simulink model "PID_time_scale_sep"  (R2023b)
settings: Solver=VariableStepAuto  StartTime=0.0  StopTime=2000  RelTol=1e-3
values from neighbouring files (symbols this model uses):
  beta = 40*pi/180    (= 0.698131700798)    [init_PID_time_scale_sep.m]
  H_c_max = 0.035    [init_PID_time_scale_sep.m]
  I = [2.10, 0, 0; 0, 2.3, -0.03; 0.01, -0.03, 1.72]    [init_PID_time_scale_sep.m]
  I_inv = inv(I)    [init_PID_time_scale_sep.m]
  K_redist = [1;1;5]*1e0    [init_PID_time_scale_sep.m]
  K_unload = 1.5*[1;1;1]*1e2    [init_PID_time_scale_sep.m]
  Kd_t = 2*1e-4    (= 0.0002)    [init_PID_time_scale_sep.m]
  Kd_w = 1e-1    (= 0.1)    [init_PID_time_scale_sep.m]
  Ki_t = [1;1;10]*1e-8    [init_PID_time_scale_sep.m]
  Ki_w = 0  *1e-4    (= 0)    [init_PID_time_scale_sep.m]
  Kp_t = [1;1;1]*1e-2    [init_PID_time_scale_sep.m]
  Kp_w = 1.1*[1;1 ;1]*1e-1    [init_PID_time_scale_sep.m]
  n = sqrt(mu/R^3)    [init_PID_time_scale_sep.m]
  Omega_des = [0.2,0.2,0.2].'*pi/180*0    [init_PID_time_scale_sep.m]
  Omega_i = [15    , -15, 15].'*pi/180    [init_PID_time_scale_sep.m]
  p1 = pi    (= 3.14159265359)    [init_PID_time_scale_sep.m]
  p2 = pi/2    (= 1.57079632679)    [init_PID_time_scale_sep.m]
  p3 = pi/4    (= 0.785398163397)    [init_PID_time_scale_sep.m]
  R_rw = [cos(beta), 0, -cos(beta), 0 ... (first row only)    [init_PID_time_scale_sep.m]
  R_rw_pinv = pinv(R_rw)    [init_PID_time_scale_sep.m]
  T_c_max = 0.015    [init_PID_time_scale_sep.m]
  T_d = 1e-6    (= 1e-06)    [init_PID_time_scale_sep.m]
  Theta_des = [30,50,70].'*pi/180    [init_PID_time_scale_sep.m]
  Theta_i = [0,0,0].'    [init_PID_time_scale_sep.m]
libraries: matrix_library x2
settings Model: Creator=subhechha  LastModifiedBy=subhechha

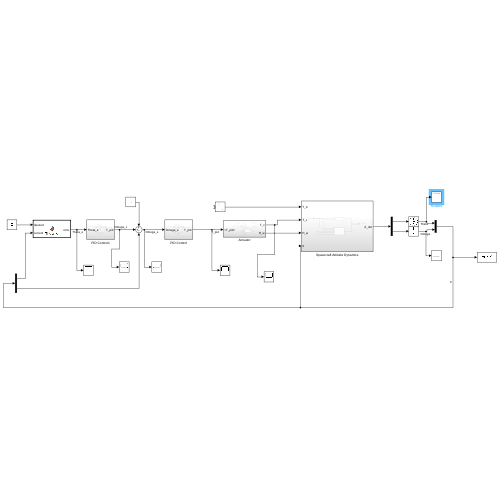
[thumbnail: Simulink's stored preview of the top-level diagram]
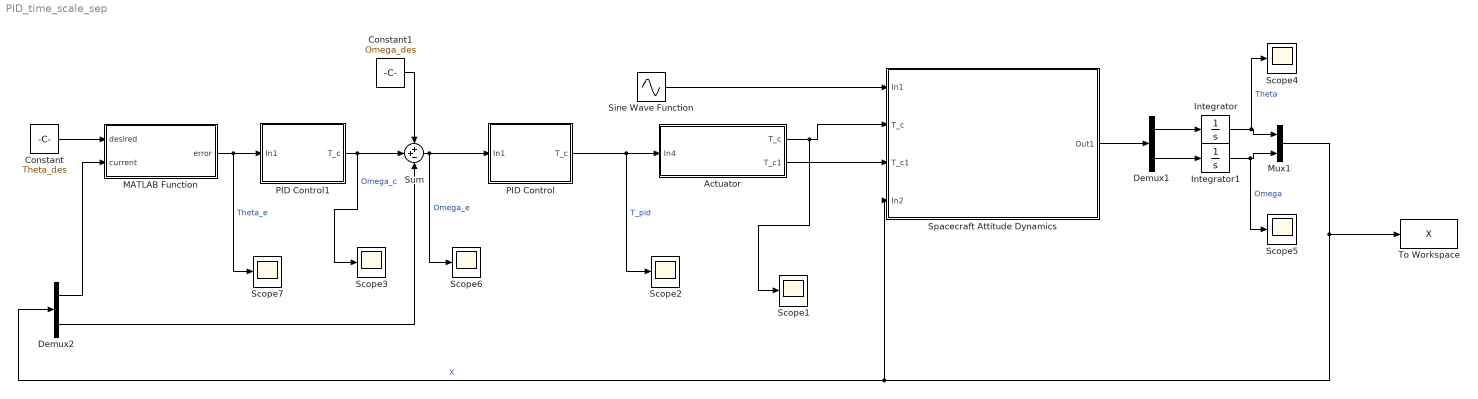
== system PID_time_scale_sep ==
  Actuator : Subsystem
  Constant : Constant  Value=Theta_des  VectorParams1D=off
  Constant1 : Constant  Value=Omega_des  VectorParams1D=off
  Demux1 : Demux  Outputs=[3 3]
  Demux2 : Demux  Outputs=[3 3]
  Integrator : Integrator  InitialCondition=Theta_i  WrapState=on  ZeroCross=off
  Integrator1 : Integrator  InitialCondition=Omega_i  ZeroCross=off
  MATLAB Function : MATLAB Function  TreatAsAtomicUnit=on
  Mux1 : Mux  Inputs=[3 3]
  PID Control : Subsystem
  PID Control1 : Subsystem
  Scope{1..7} (7 alike) : Scope
  Sine Wave Function : Sin  TimeSource=Use external signal  Amplitude=[T_d;T_d;T_d]  Frequency=0.01  Phase=[p1;p2;p3]  SampleTime=0
  Spacecraft Attitude Dynamics : Subsystem
  Sum : Sum  Inputs=++-
  To Workspace : ToWorkspace  VariableName=X  SaveFormat=Timeseries  SampleTime=-1
  wires:
  Sum/1 -> PID Control/1(In1), Scope6/1  "Omega_e"
  Actuator/1(T_c) -> Scope1/1, Spacecraft Attitude Dynamics/2(T_c)
  Actuator/2(T_c1) -> Spacecraft Attitude Dynamics/3(T_c1)
  PID Control/1(T_c) -> Scope2/1, Actuator/1(In4)  "T_pid"
  Sine Wave Function/1 -> Spacecraft Attitude Dynamics/1(In1)
  Demux1/2 -> Integrator1/1
  Demux1/1 -> Integrator/1
  Spacecraft Attitude Dynamics/1(Out1) -> Demux1/1
  Mux1/1 -> Demux2/1, Spacecraft Attitude Dynamics/4(In2), To Workspace/1  "X"
  Integrator1/1 -> Scope5/1, Mux1/2  "Omega"
  Integrator/1 -> Scope4/1, Mux1/1  "Theta"
  Demux2/2 -> Sum/3
  PID Control1/1(T_c) -> Sum/2, Scope3/1  "Omega_c"
  MATLAB Function/1(error) -> Scope7/1, PID Control1/1(In1)  "Theta_e"
  Demux2/1 -> MATLAB Function/2(current)
  Constant/1 -> MATLAB Function/1(desired)
  Constant1/1 -> Sum/1

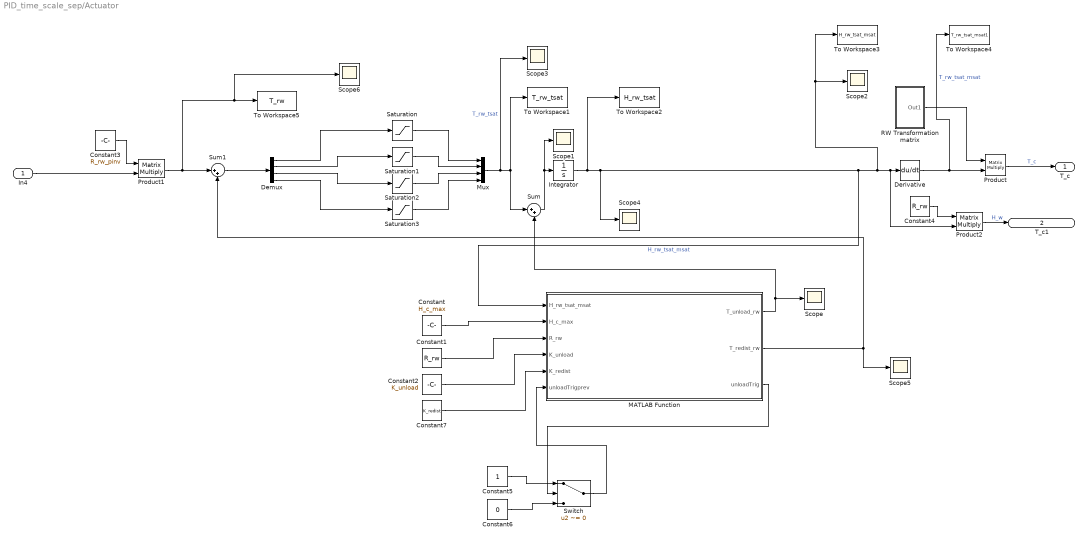
== system PID_time_scale_sep/Actuator ==
  In4 : Inport
  Constant : Constant  Value=H_c_max
  Constant1 : Constant  Value=R_rw  VectorParams1D=off
  Constant2 : Constant  Value=K_unload  VectorParams1D=off
  Constant3 : Constant  Value=R_rw_pinv  VectorParams1D=off
  Constant4 : Constant  Value=R_rw  VectorParams1D=off
  Constant5 : Constant
  Constant6 : Constant  Value=0
  Constant7 : Constant  Value=K_redist  VectorParams1D=off
  Demux : Demux
  Derivative : Derivative
  Integrator : Integrator  LimitOutput=on  UpperSaturationLimit=H_c_max  LowerSaturationLimit=-H_c_max  ZeroCross=off
  MATLAB Function : MATLAB Function  TreatAsAtomicUnit=on
  Mux : Mux
  Product : Product  Multiplication=Matrix(*)
  Product1 : Product  Multiplication=Matrix(*)
  Product2 : Product  Multiplication=Matrix(*)
  RW Transformation matrix : Subsystem
  Saturation{,1..3} (4 alike) : Saturate  UpperLimit=T_c_max  LowerLimit=-T_c_max  LinearizeAsGain=off  ZeroCross=off
  Scope{,1..6} (7 alike) : Scope
  Sum : Sum  Inputs=|++
  Sum1 : Sum  Inputs=|++
  Switch : Switch  Criteria=u2 ~= 0  SaturateOnIntegerOverflow=off  InputSameDT=off
  To Workspace1 : ToWorkspace  VariableName=T_rw_tsat  SaveFormat=Timeseries  SampleTime=-1
  To Workspace2 : ToWorkspace  VariableName=H_rw_tsat  SaveFormat=Timeseries  SampleTime=-1
  To Workspace3 : ToWorkspace  VariableName=H_rw_tsat_msat  SaveFormat=Timeseries  SampleTime=-1
  To Workspace4 : ToWorkspace  VariableName=T_rw_tsat_msat1  SaveFormat=Timeseries  SampleTime=-1
  To Workspace5 : ToWorkspace  VariableName=T_rw  SaveFormat=Timeseries  SampleTime=-1
  T_c : Outport
  T_c1 : Outport  Port=2
  wires:
  Mux/1 -> Scope3/1, To Workspace1/1, Sum/1  "T_rw_tsat"
  Demux/3 -> Saturation2/1
  Demux/2 -> Saturation1/1
  Saturation/1 -> Mux/1
  Saturation3/1 -> Mux/4
  Integrator/1 -> To Workspace2/1, MATLAB Function/1(H_rw_tsat_msat), Product2/2, Derivative/1, Scope2/1, To Workspace3/1, Scope4/1  "H_rw_tsat_msat"
  Saturation1/1 -> Mux/2
  Product1/1 -> Sum1/1, Scope6/1, To Workspace5/1
  Saturation2/1 -> Mux/3
  Demux/1 -> Saturation/1
  Derivative/1 -> To Workspace4/1, Product/2  "T_rw_tsat_msat"
  Demux/4 -> Saturation3/1
  RW Transformation matrix/1(Out1) -> Product/1
  Product/1 -> T_c/1  "T_c"
  Constant/1 -> MATLAB Function/2(H_c_max)
  Constant1/1 -> MATLAB Function/3(R_rw)
  Constant2/1 -> MATLAB Function/4(K_unload)
  In4/1 -> Product1/2
  Constant3/1 -> Product1/1
  Sum/1 -> Scope1/1, Integrator/1
  MATLAB Function/1(T_unload_rw) -> Sum/2, Scope/1
  Product2/1 -> T_c1/1  "H_w"
  Constant4/1 -> Product2/1
  MATLAB Function/3(unloadTrig) -> Switch/2
  Switch/1 -> MATLAB Function/6(unloadTrigprev)
  Constant5/1 -> Switch/1
  Constant6/1 -> Switch/3
  Constant7/1 -> MATLAB Function/5(K_redist)
  MATLAB Function/2(T_redist_rw) -> Sum1/2, Scope5/1
  Sum1/1 -> Demux/1

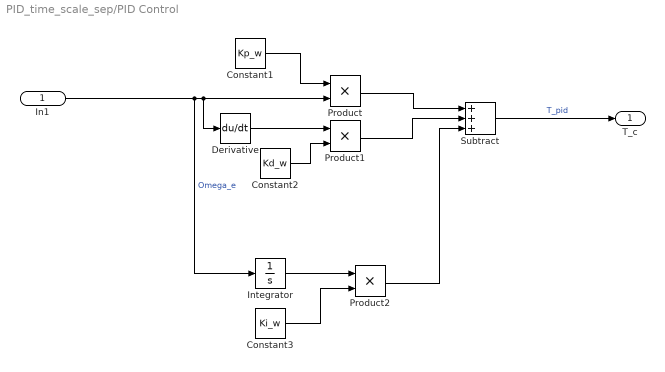
== system PID_time_scale_sep/PID Control ==
  In1 : Inport
  Constant1 : Constant  Value=Kp_w  VectorParams1D=off
  Constant2 : Constant  Value=Kd_w  VectorParams1D=off
  Constant3 : Constant  Value=Ki_w  VectorParams1D=off
  Derivative : Derivative
  Integrator : Integrator  WrapState=on
  Product : Product
  Product1 : Product
  Product2 : Product
  Subtract : Sum  Inputs=+++
  T_c : Outport
  wires:
  Constant2/1 -> Product1/2
  Product1/1 -> Subtract/2
  Constant1/1 -> Product/1
  Product/1 -> Subtract/1
  Subtract/1 -> T_c/1  "T_pid"
  Integrator/1 -> Product2/1
  Constant3/1 -> Product2/2
  Product2/1 -> Subtract/3
  In1/1 -> Integrator/1, Derivative/1, Product/2  "Omega_e"
  Derivative/1 -> Product1/1

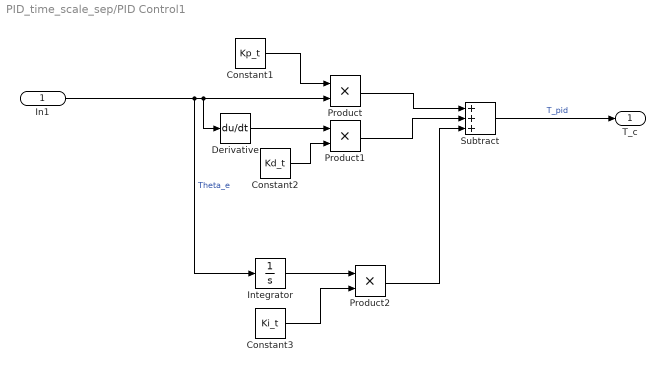
== system PID_time_scale_sep/PID Control1 ==
  In1 : Inport
  Constant1 : Constant  Value=Kp_t  VectorParams1D=off
  Constant2 : Constant  Value=Kd_t  VectorParams1D=off
  Constant3 : Constant  Value=Ki_t  VectorParams1D=off
  Derivative : Derivative
  Integrator : Integrator  WrapState=on
  Product : Product
  Product1 : Product
  Product2 : Product
  Subtract : Sum  Inputs=+++
  T_c : Outport
  wires:
  Constant2/1 -> Product1/2
  Product1/1 -> Subtract/2
  Constant1/1 -> Product/1
  Product/1 -> Subtract/1
  Subtract/1 -> T_c/1  "T_pid"
  Integrator/1 -> Product2/1
  Constant3/1 -> Product2/2
  Product2/1 -> Subtract/3
  In1/1 -> Integrator/1, Derivative/1, Product/2  "Theta_e"
  Derivative/1 -> Product1/1

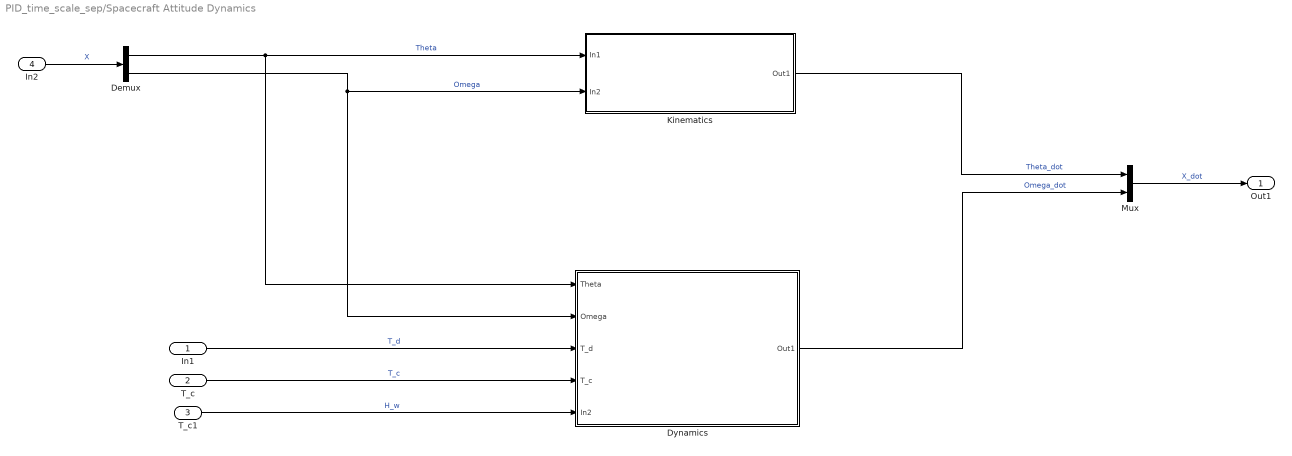
== system PID_time_scale_sep/Spacecraft Attitude Dynamics ==
  In1 : Inport
  T_c : Inport  Port=2
  T_c1 : Inport  Port=3
  In2 : Inport  Port=4
  Demux : Demux  Outputs=[3 3]
  Dynamics : Subsystem
  Kinematics : Subsystem
  Mux : Mux  Inputs=[3 3]
  Out1 : Outport
  wires:
  Dynamics/1(Out1) -> Mux/2  "Omega_dot"
  Kinematics/1(Out1) -> Mux/1  "Theta_dot"
  Demux/1 -> Dynamics/1(Theta), Kinematics/1(In1)  "Theta"
  In1/1 -> Dynamics/3(T_d)  "T_d"
  Demux/2 -> Dynamics/2(Omega), Kinematics/2(In2)  "Omega"
  In2/1 -> Demux/1  "X"
  Mux/1 -> Out1/1  "X_dot"
  T_c/1 -> Dynamics/4(T_c)  "T_c"
  T_c1/1 -> Dynamics/5(In2)  "H_w"

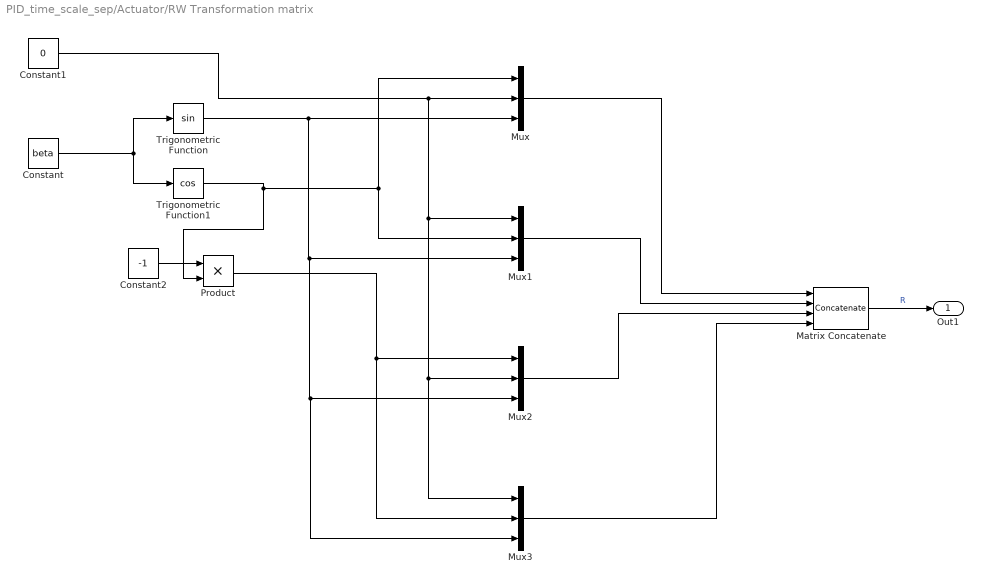
== system PID_time_scale_sep/Actuator/RW Transformation matrix ==
  Constant : Constant  Value=beta
  Constant1 : Constant  Value=0
  Constant2 : Constant  Value=-1
  Matrix Concatenate : Concatenate  NumInputs=4  Mode=Multidimensional array  ConcatenateDimension=2
  Mux{,1..3} (4 alike) : Mux  Inputs=3
  Product : Product
  Trigonometric Function : Trigonometry
  Trigonometric Function1 : Trigonometry  Operator=cos
  Out1 : Outport
  wires:
  Mux3/1 -> Matrix Concatenate/4
  Constant2/1 -> Product/1
  Product/1 -> Mux3/2, Mux2/1
  Mux/1 -> Matrix Concatenate/1
  Trigonometric Function1/1 -> Mux/1, Mux1/2, Product/2
  Mux1/1 -> Matrix Concatenate/2
  Mux2/1 -> Matrix Concatenate/3
  Constant/1 -> Trigonometric Function1/1, Trigonometric Function/1
  Trigonometric Function/1 -> Mux3/3, Mux2/3, Mux1/3, Mux/3
  Constant1/1 -> Mux3/1, Mux2/2, Mux1/1, Mux/2
  Matrix Concatenate/1 -> Out1/1  "R"

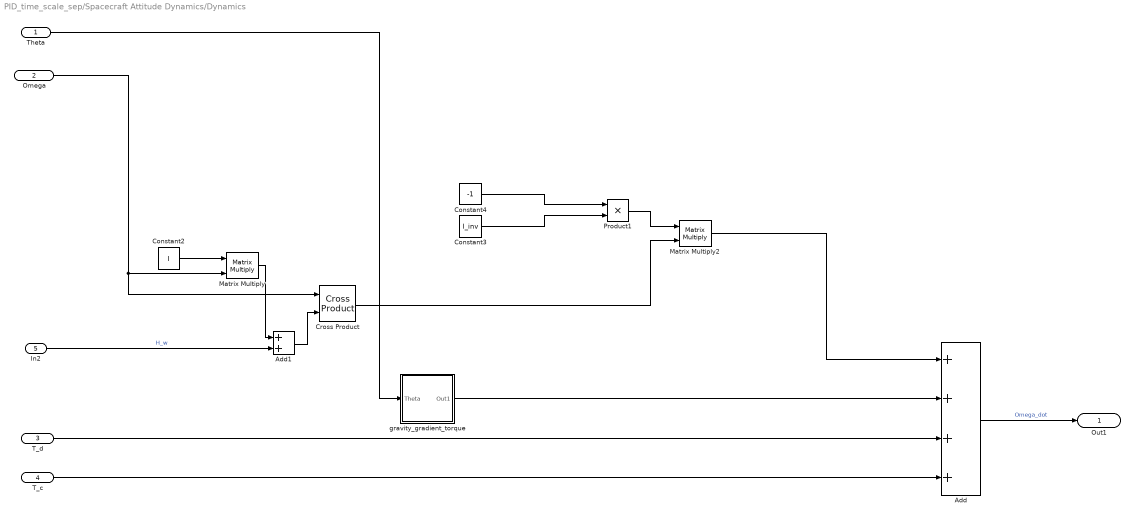
== system PID_time_scale_sep/Spacecraft Attitude Dynamics/Dynamics ==
  Theta : Inport
  Omega : Inport  Port=2
  T_d : Inport  Port=3
  T_c : Inport  Port=4
  In2 : Inport  Port=5
  Add : Sum  Inputs=++++
  Add1 : Sum
  Constant2 : Constant  Value=I  VectorParams1D=off
  Constant3 : Constant  Value=I_inv  VectorParams1D=off
  Constant4 : Constant  Value=-1
  Cross Product : matrix_library/Cross Product
  Matrix Multiply : Product  Multiplication=Matrix(*)
  Matrix Multiply2 : Product  Multiplication=Matrix(*)
  Product1 : Product
  gravity_gradient_torque : Subsystem
  Out1 : Outport
  wires:
  Add/1 -> Out1/1  "Omega_dot"
  T_c/1 -> Add/4
  Matrix Multiply/1 -> Add1/1
  T_d/1 -> Add/3
  Theta/1 -> gravity_gradient_torque/1(Theta)
  Constant4/1 -> Product1/1
  Matrix Multiply2/1 -> Add/1
  Product1/1 -> Matrix Multiply2/1
  Constant2/1 -> Matrix Multiply/1
  Constant3/1 -> Product1/2
  Cross Product/1 -> Matrix Multiply2/2
  Omega/1 -> Cross Product/1, Matrix Multiply/2
  gravity_gradient_torque/1(Out1) -> Add/2
  In2/1 -> Add1/2  "H_w"
  Add1/1 -> Cross Product/2

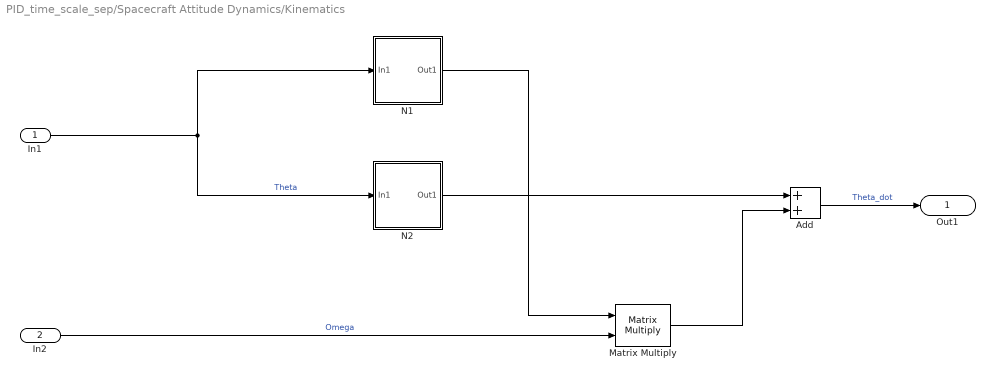
== system PID_time_scale_sep/Spacecraft Attitude Dynamics/Kinematics ==
  In1 : Inport
  In2 : Inport  Port=2
  Add : Sum
  Matrix Multiply : Product  Multiplication=Matrix(*)
  N1 : Subsystem
  N2 : Subsystem
  Out1 : Outport
  wires:
  N2/1(Out1) -> Add/1
  In1/1 -> N1/1(In1), N2/1(In1)  "Theta"
  Matrix Multiply/1 -> Add/2
  N1/1(Out1) -> Matrix Multiply/1
  Add/1 -> Out1/1  "Theta_dot"
  In2/1 -> Matrix Multiply/2  "Omega"

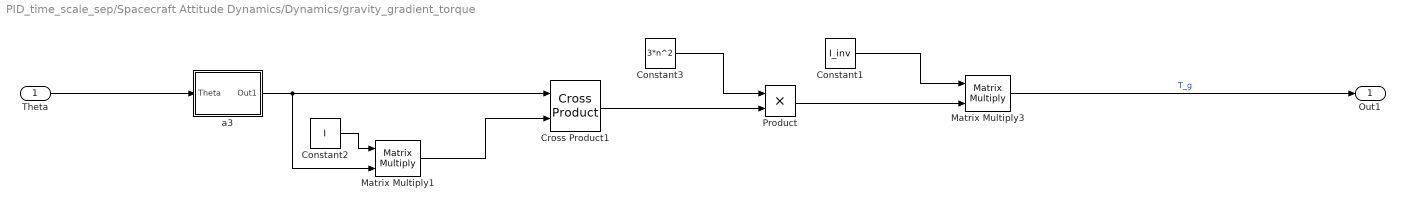
== system PID_time_scale_sep/Spacecraft Attitude Dynamics/Dynamics/gravity_gradient_torque ==
  Theta : Inport
  Constant1 : Constant  Value=I_inv  VectorParams1D=off
  Constant2 : Constant  Value=I  VectorParams1D=off
  Constant3 : Constant  Value=3*n^2  VectorParams1D=off
  Cross Product1 : matrix_library/Cross Product
  Matrix Multiply1 : Product  Multiplication=Matrix(*)
  Matrix Multiply3 : Product  Multiplication=Matrix(*)
  Product : Product
  a3 : Subsystem
  Out1 : Outport
  wires:
  Matrix Multiply1/1 -> Cross Product1/2
  Constant3/1 -> Product/1
  a3/1(Out1) -> Cross Product1/1, Matrix Multiply1/2
  Product/1 -> Matrix Multiply3/2
  Cross Product1/1 -> Product/2
  Matrix Multiply3/1 -> Out1/1  "T_g"
  Theta/1 -> a3/1(Theta)
  Constant1/1 -> Matrix Multiply3/1
  Constant2/1 -> Matrix Multiply1/1

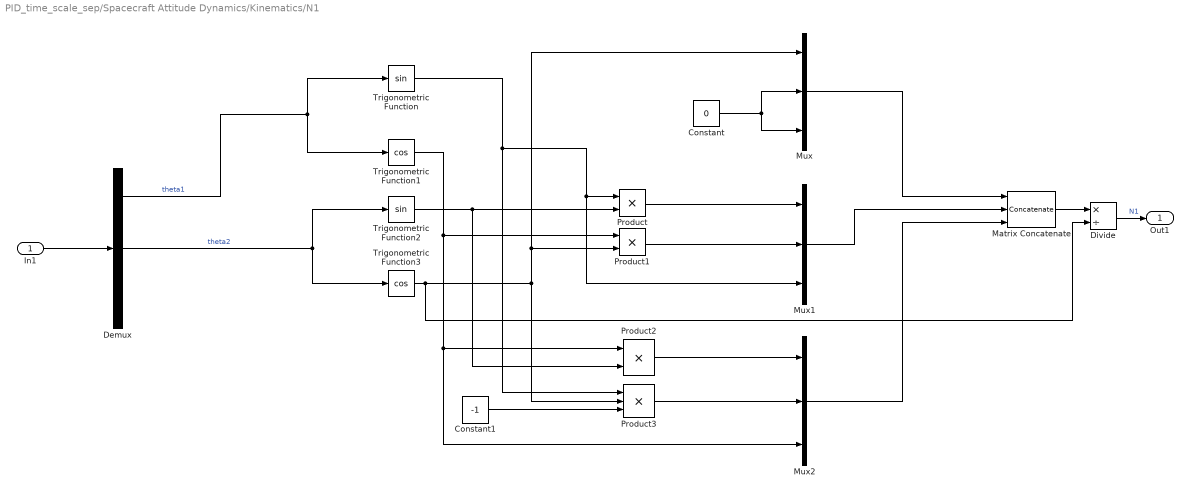
== system PID_time_scale_sep/Spacecraft Attitude Dynamics/Kinematics/N1 ==
  In1 : Inport
  Constant : Constant  Value=0
  Constant1 : Constant  Value=-1
  Demux : Demux  Outputs=3
  Divide : Product  Inputs=*/
  Matrix Concatenate : Concatenate  NumInputs=3  Mode=Multidimensional array  ConcatenateDimension=2
  Mux : Mux  Inputs=3
  Mux1 : Mux  Inputs=3
  Mux2 : Mux  Inputs=3
  Product : Product
  Product1 : Product
  Product2 : Product
  Product3 : Product  Inputs=3
  Trigonometric Function : Trigonometry
  Trigonometric Function1 : Trigonometry  Operator=cos
  Trigonometric Function2 : Trigonometry
  Trigonometric Function3 : Trigonometry  Operator=cos
  Out1 : Outport
  wires:
  In1/1 -> Demux/1
  Matrix Concatenate/1 -> Divide/1
  Constant1/1 -> Product3/3
  Product/1 -> Mux1/1
  Demux/2 -> Trigonometric Function3/1, Trigonometric Function2/1  "theta2"
  Mux1/1 -> Matrix Concatenate/2
  Constant/1 -> Mux/3, Mux/2
  Trigonometric Function/1 -> Product3/1, Mux1/3, Product/1
  Mux2/1 -> Matrix Concatenate/3
  Product1/1 -> Mux1/2
  Trigonometric Function3/1 -> Divide/2, Product3/2, Mux/1, Product1/2
  Product3/1 -> Mux2/2
  Demux/1 -> Trigonometric Function1/1, Trigonometric Function/1  "theta1"
  Mux/1 -> Matrix Concatenate/1
  Product2/1 -> Mux2/1
  Trigonometric Function1/1 -> Mux2/3, Product2/1, Product1/1
  Trigonometric Function2/1 -> Product2/2, Product/2
  Divide/1 -> Out1/1  "N1"

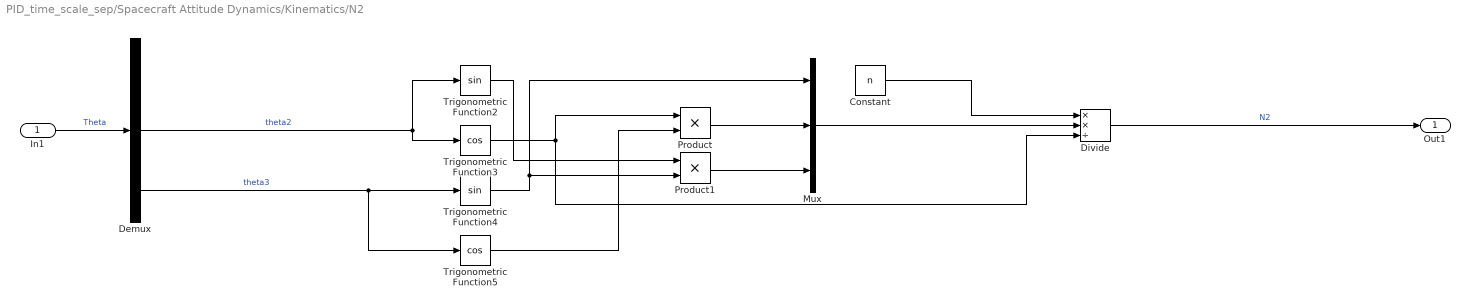
== system PID_time_scale_sep/Spacecraft Attitude Dynamics/Kinematics/N2 ==
  In1 : Inport
  Constant : Constant  Value=n
  Demux : Demux  Outputs=3
  Divide : Product  Inputs=**/
  Mux : Mux  Inputs=3
  Product : Product
  Product1 : Product
  Trigonometric Function2 : Trigonometry
  Trigonometric Function3 : Trigonometry  Operator=cos
  Trigonometric Function4 : Trigonometry
  Trigonometric Function5 : Trigonometry  Operator=cos
  Out1 : Outport
  wires:
  In1/1 -> Demux/1  "Theta"
  Demux/2 -> Trigonometric Function2/1, Trigonometric Function3/1  "theta2"
  Trigonometric Function4/1 -> Product1/2, Mux/1
  Demux/3 -> Trigonometric Function5/1, Trigonometric Function4/1  "theta3"
  Trigonometric Function3/1 -> Divide/3, Product/1
  Trigonometric Function5/1 -> Product/2
  Product/1 -> Mux/2
  Product1/1 -> Mux/3
  Constant/1 -> Divide/1
  Mux/1 -> Divide/2
  Divide/1 -> Out1/1  "N2"
  Trigonometric Function2/1 -> Product1/1

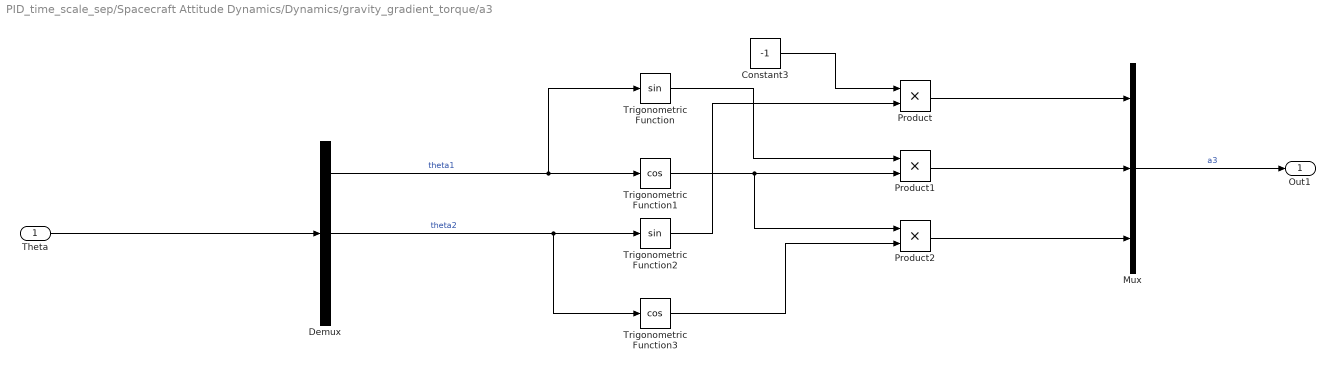
== system PID_time_scale_sep/Spacecraft Attitude Dynamics/Dynamics/gravity_gradient_torque/a3 ==
  Theta : Inport
  Constant3 : Constant  Value=-1
  Demux : Demux  Outputs=3
  Mux : Mux  Inputs=3
  Product : Product
  Product1 : Product
  Product2 : Product
  Trigonometric Function : Trigonometry
  Trigonometric Function1 : Trigonometry  Operator=cos
  Trigonometric Function2 : Trigonometry
  Trigonometric Function3 : Trigonometry  Operator=cos
  Out1 : Outport
  wires:
  Trigonometric Function2/1 -> Product/2
  Product2/1 -> Mux/3
  Trigonometric Function3/1 -> Product2/2
  Product/1 -> Mux/1
  Product1/1 -> Mux/2
  Trigonometric Function/1 -> Product1/1
  Demux/2 -> Trigonometric Function3/1, Trigonometric Function2/1  "theta2"
  Constant3/1 -> Product/1
  Trigonometric Function1/1 -> Product2/1, Product1/2
  Demux/1 -> Trigonometric Function/1, Trigonometric Function1/1  "theta1"
  Theta/1 -> Demux/1
  Mux/1 -> Out1/1  "a3"

== matlab function PID_time_scale_sep/MATLAB Function ==
  data: desired input; current input; error output
function error = Theta_e(desired, current)
    error = mod(desired - current + pi, 2*pi) - pi;
end

== matlab function PID_time_scale_sep/Actuator/MATLAB Function ==
  data: H_rw_tsat_msat input; T_unload_rw output; T_redist_rw output; H_c_max input; R_rw input; K_unload input; K_redist input; unloadTrigprev input; unloadTrig output
function [T_unload_rw, T_redist_rw,unloadTrig] = momentum_manage(H_rw_tsat_msat,H_c_max, R_rw, K_unload,K_redist,unloadTrigprev)
% Specify output sizes
%coder.outputsize(T_unload, [3,1]);  % output1 is a 3x1 vector
%coder.outputsize(output2, [4,4]);  % output2 is a 4x4 matrix
%disp(unloadTrigprev)
% Safety threshold for unloading (e.g., 90% of H_max)
% unloadTrigprev=0;
threshold_redist = 0.8 * H_c_max;
threshold_unload = 0.8*4*H_c_max;
unload_complete = 0.1*4*H_c_max;

%H_body = R_rw*H_rw_tsat_msat;
H_total = sum(abs(H_rw_tsat_msat));
T_unload = zeros(3,1);
T_redist = zeros(3,1);
T_unload_rw=zeros(size(H_rw_tsat_msat));
T_redist_rw=zeros(size(H_rw_tsat_msat));

% Check if any wheel exceeds the threshold
triggerRedist = any(abs(H_rw_tsat_msat) > threshold_redist);


% Check if total momentum exceeds unloading threshold
triggerUnloadStart = H_total > threshold_unload;

H_desired_rw=zeros(size(H_rw_tsat_msat));
% fprintf('previous trigger in unload loop %f \n', unloadTrigprev);
%fprintf('unload %f redist %s\n',unloadTrigprev,string(triggerRedist));
if (triggerUnloadStart | unloadTrigprev)
    % Unloading mode
    fprintf('unload %f %f \n',H_total,unload_complete);
    unloadTrig=1;
    if H_total<unload_complete
        unloadTrig=0;
    end
    H_desired_rw = 0.1*H_c_max*ones(4, 1);  % Aim to reduce total momentum to zero
    T_unload = -K_unload .* (R_rw*(H_rw_tsat_msat - H_desired_rw));

elseif triggerRedist & (~unloadTrigprev)
    unloadTrig=unloadTrigprev;
    % fprintf('redist %f \n',H_total);
    m_factor = zeros(1,4);
    for i=1:length(H_rw_tsat_msat)
        if abs(H_rw_tsat_msat(i))>threshold_redist
            H_desired_rw(i)=0;
            m_factor(i)=0;
        else
            H_desired_rw(i)=H_rw_tsat_msat(i);
            m_factor(i)=1;
        end
    end
    del_H_rw = (H_rw_tsat_msat-H_desired_rw);
    del_H = R_rw*del_H_rw;
    H_redist = pinv(R_rw.*m_factor)*del_H;
    H_desired_redist_rw = H_desired_rw+H_redist;
    % RH_desired = R_rw*H_desired_rw;
    T_redist = -K_redist.*(R_rw*(H_rw_tsat_msat-H_desired_rw));
else
    unloadTrig=unloadTrigprev;
end
T_unload_rw = pinv(R_rw)*T_unload;
T_redist_rw = pinv(R_rw)*T_redist;
end
